simulink model "state_observer_2023b"  (R2023b)
settings: Solver=VariableStepAuto  StartTime=0.0  StopTime=10.0  RelTol=1e-3
undefined symbols (not defined in the file): b, J, K, Kc, L, Lc, R
settings Model: Creator=Harish  LastModifiedBy=Harish
settings RTWCC: GPUComputeCapability=5.0

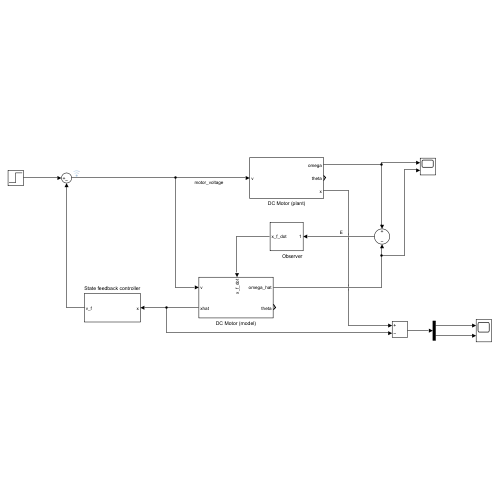
[thumbnail: Simulink's stored preview of the top-level diagram]
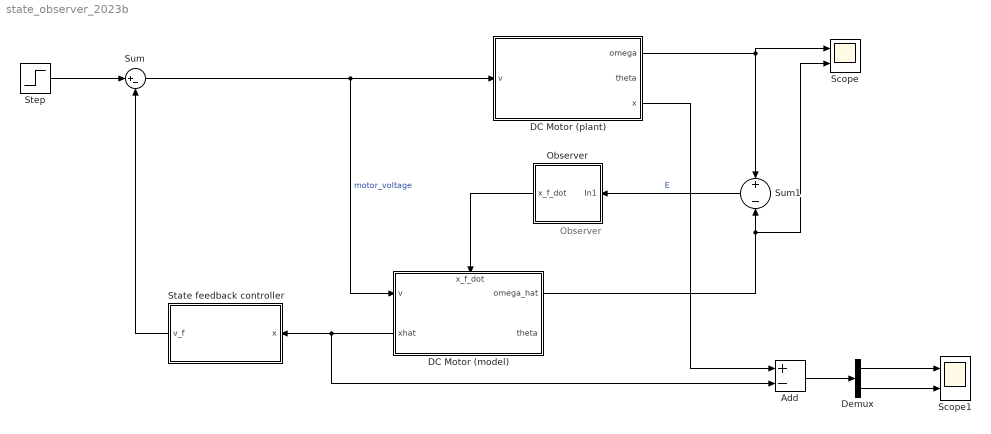
== system state_observer_2023b ==
  note: Observer
  Add : Sum  Inputs=+-
  DC Motor (model) : Subsystem
      settings: PortSchema="{\"entries\":[{\"content\":{\"sides\":[{\"content\":{\"connectorIds\":[\"In1\",\"Out3\"]},\"type\":\"ConnectorPlacement.EquallySpacedRectSide\",\"uuid\":\"2b483e04-f0bf-4587-962d-f1e1055a504f\"},{\"content\":{\"connectorIds\":[\"Out1\",\"Out2\"],\"side\":\"RIGHT\"},\"type\":\"ConnectorPlacement.EquallySpacedRectSide\",\"uuid\":\"def1afe8-227d-4da8-931b-63cfceb9275c\"},{\"content\":{\"connectorIds\":[\"In2\"],\"side\":\"TOP\"},\"type\":\"ConnectorPlacement.EquallySpacedRectSide\",\"uuid\":\"83491253-a60e-40c0-9750-a91f8b421144\"}]},\"type\":\"ConnectorPlacement.EquallySpacedConnector\",\"uuid\":\"4f5576a8-263a-420b-867e-94d06ccc103a\"}],\"packageUris\":[\"http://schema.mathworks.com/mf0/Connector/R2020b\"],\"version\":\"1.0\"}"
  DC Motor (plant) : Subsystem
  Demux : Demux  Outputs=2
  Observer : Subsystem
  Scope : Scope  NumInputPorts=2
  Scope1 : Scope  NumInputPorts=2
  State feedback controller : Subsystem
  Step : Step  SampleTime=0
  Sum : Sum  Inputs=|+-
  Sum1 : Sum  Inputs=+|-
  wires:
  Sum/1 -> DC Motor (model)/1(v), DC Motor (plant)/1(v)  "motor_voltage"
  DC Motor (plant)/1(omega) -> Scope/1, Sum1/1
  Step/1 -> Sum/1
  DC Motor (model)/1(omega_hat) -> Scope/2, Sum1/2
  Sum1/1 -> Observer/1(In1)  "E"
  Observer/1(x_f_dot) -> DC Motor (model)/2(x_f_dot)
  DC Motor (model)/3(xhat) -> Add/2, State feedback controller/1(x)
  State feedback controller/1(v_f) -> Sum/2
  DC Motor (plant)/3(x) -> Add/1
  Add/1 -> Demux/1
  Demux/1 -> Scope1/1
  Demux/2 -> Scope1/2

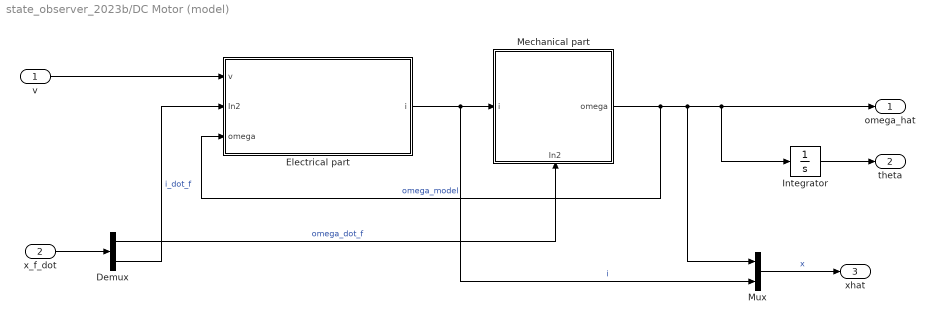
== system state_observer_2023b/DC Motor (model) ==
  v : Inport
  x_f_dot : Inport  Port=2
  Demux : Demux  Outputs=2
  "Electrical part " : Subsystem
  Integrator : Integrator
  Mechanical part : Subsystem
      settings: PortSchema="{\"entries\":[{\"content\":{\"sides\":[{\"content\":{\"connectorIds\":[\"In1\"]},\"type\":\"ConnectorPlacement.EquallySpacedRectSide\",\"uuid\":\"cfa22e76-426c-462d-8ef8-59579940fa0d\"},{\"content\":{\"connectorIds\":[\"Out1\"],\"side\":\"RIGHT\"},\"type\":\"ConnectorPlacement.EquallySpacedRectSide\",\"uuid\":\"d76cab75-f381-41dd-b31a-a9854dc13879\"},{\"content\":{\"side\":\"TOP\"},\"type\":\"ConnectorPlacement.EquallySpacedRectSide\",\"uuid\":\"0693442b-bae3-4156-915c-17f4d78fd8df\"},{\"content\":{\"connectorIds\":[\"In2\"],\"side\":\"BOTTOM\"},\"type\":\"ConnectorPlacement.EquallySpacedRectSide\",\"uuid\":\"c4b3b7a3-04e2-4e42-8ee1-dd16592de4f8\"}]},\"type\":\"ConnectorPlacement.EquallySpacedConnector\",\"uuid\":\"090e9602-d875-46fe-83df-94f978736a7a\"}],\"packageUris\":[\"http://schema.mathworks.com/mf0/Connector/R2020b\"],\"version\":\"1.0\"}"
  Mux : Mux  Inputs=2
  omega_hat : Outport
  theta : Outport  Port=2
  xhat : Outport  Port=3
  wires:
  Mux/1 -> xhat/1  "x"
  Integrator/1 -> theta/1
  v/1 -> "Electrical part "/1(v)
  Mechanical part/1(omega) -> "Electrical part "/3(omega), omega_hat/1, Integrator/1, Mux/1  "omega_model"
  "Electrical part "/1(i) -> Mechanical part/1(i), Mux/2  "i"
  x_f_dot/1 -> Demux/1
  Demux/1 -> Mechanical part/2(In2)  "omega_dot_f"
  Demux/2 -> "Electrical part "/2(In2)  "i_dot_f"

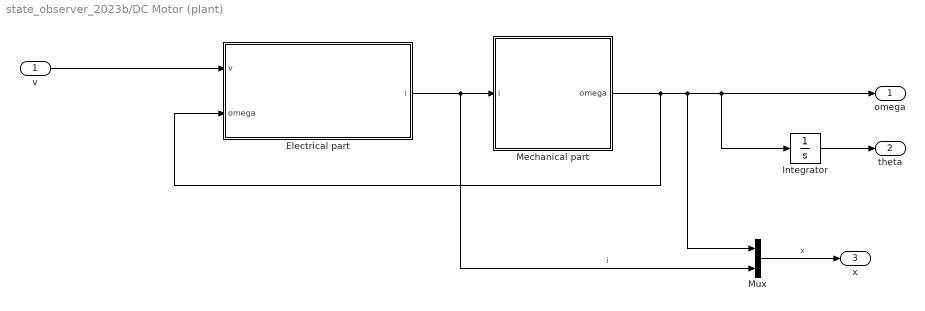
== system state_observer_2023b/DC Motor (plant) ==
  v : Inport
  "Electrical part " : Subsystem
  Integrator : Integrator
  Mechanical part : Subsystem
  Mux : Mux  Inputs=2
  omega : Outport
  theta : Outport  Port=2
  x : Outport  Port=3
  wires:
  "Electrical part "/1(i) -> Mux/2, Mechanical part/1(i)  "i"
  Mechanical part/1(omega) -> Mux/1, Integrator/1, omega/1, "Electrical part "/2(omega)
  v/1 -> "Electrical part "/1(v)
  Integrator/1 -> theta/1
  Mux/1 -> x/1  "x"

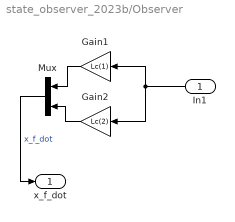
== system state_observer_2023b/Observer ==
  In1 : Inport
  Gain1 : Gain  Gain=Lc(1)
  Gain2 : Gain  Gain=Lc(2)
  Mux : Mux  Inputs=2
  x_f_dot : Outport
  wires:
  Gain2/1 -> Mux/2
  Gain1/1 -> Mux/1
  In1/1 -> Gain2/1, Gain1/1
  Mux/1 -> x_f_dot/1  "x_f_dot"

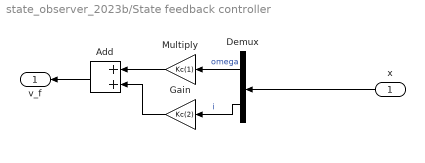
== system state_observer_2023b/State feedback controller ==
  x : Inport
  Add : Sum
  Demux : Demux  Outputs=2
  Gain : Gain  Gain=Kc(2)
  Multiply : Gain  Gain=Kc(1)
  v_f : Outport
  wires:
  x/1 -> Demux/1
  Multiply/1 -> Add/1
  Add/1 -> v_f/1
  Demux/1 -> Multiply/1  "omega"
  Demux/2 -> Gain/1  "i"
  Gain/1 -> Add/2

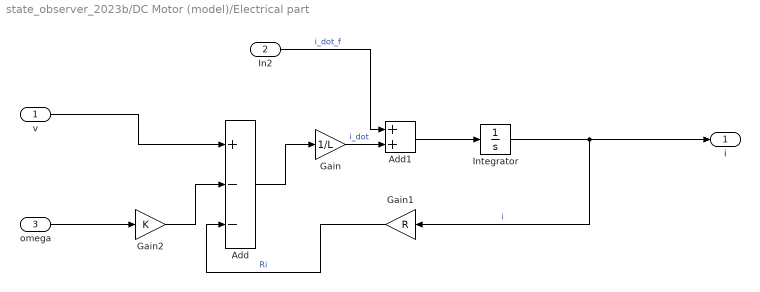
== system state_observer_2023b/DC Motor (model)/Electrical part  ==
  v : Inport
  In2 : Inport  Port=2
  omega : Inport  Port=3
  Add : Sum  Inputs=+--
  Add1 : Sum
  Gain : Gain  Gain=1/L
  Gain1 : Gain  Gain=R
  Gain2 : Gain  Gain=K
  Integrator : Integrator
  i : Outport
  wires:
  omega/1 -> Gain2/1
  Gain2/1 -> Add/2
  v/1 -> Add/1
  Gain1/1 -> Add/3  "Ri"
  Integrator/1 -> Gain1/1, i/1  "i"
  Add/1 -> Gain/1
  In2/1 -> Add1/1  "i_dot_f"
  Gain/1 -> Add1/2  "i_dot"
  Add1/1 -> Integrator/1

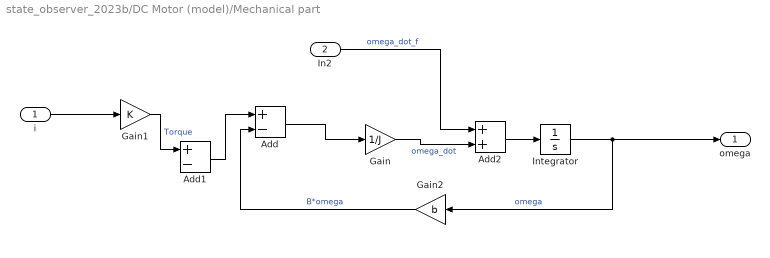
== system state_observer_2023b/DC Motor (model)/Mechanical part ==
  i : Inport
  In2 : Inport  Port=2
  Add : Sum  Inputs=+-
  Add1 : Sum  Inputs=+-
  Add2 : Sum
  Gain : Gain  Gain=1/J
  Gain1 : Gain  Gain=K
  Gain2 : Gain  Gain=b
  Integrator : Integrator
  omega : Outport
  wires:
  Add1/1 -> Add/1
  Gain1/1 -> Add1/1  "Torque"
  i/1 -> Gain1/1
  Gain2/1 -> Add/2  "B*omega"
  Integrator/1 -> Gain2/1, omega/1  "omega"
  Add/1 -> Gain/1
  In2/1 -> Add2/1  "omega_dot_f"
  Gain/1 -> Add2/2  "omega_dot"
  Add2/1 -> Integrator/1

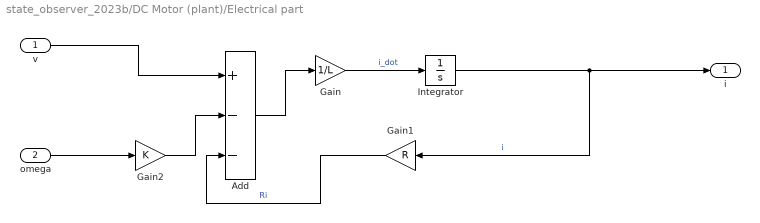
== system state_observer_2023b/DC Motor (plant)/Electrical part  ==
  v : Inport
  omega : Inport  Port=2
  Add : Sum  Inputs=+--
  Gain : Gain  Gain=1/L
  Gain1 : Gain  Gain=R
  Gain2 : Gain  Gain=K
  Integrator : Integrator  InitialCondition=0.5
  i : Outport
  wires:
  Add/1 -> Gain/1
  Integrator/1 -> i/1, Gain1/1  "i"
  Gain1/1 -> Add/3  "Ri"
  v/1 -> Add/1
  Gain2/1 -> Add/2
  Gain/1 -> Integrator/1  "i_dot"
  omega/1 -> Gain2/1

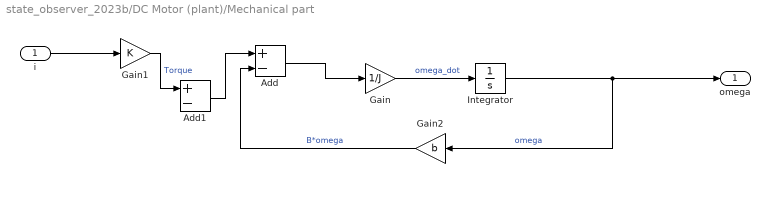
== system state_observer_2023b/DC Motor (plant)/Mechanical part ==
  i : Inport
  Add : Sum  Inputs=+-
  Add1 : Sum  Inputs=+-
  Gain : Gain  Gain=1/J
  Gain1 : Gain  Gain=K
  Gain2 : Gain  Gain=b
  Integrator : Integrator  InitialCondition=0.05
  omega : Outport
  wires:
  Add/1 -> Gain/1
  Integrator/1 -> omega/1, Gain2/1  "omega"
  Gain2/1 -> Add/2  "B*omega"
  i/1 -> Gain1/1
  Gain/1 -> Integrator/1  "omega_dot"
  Gain1/1 -> Add1/1  "Torque"
  Add1/1 -> Add/1
